simulink model "prelab1"  (R2020a)
settings: Solver=VariableStepAuto  StartTime=0.0  StopTime=10.0  RelTol=1e-3
values from neighbouring files (symbols this model uses):
  backEmfConstant = Kb    (= 0.4173)    [simplified_tf.m]    (also in transferFunctionsDef.m)
  electricalWindingOfMotor = 1/(La*s+Ra)    [simplified_tf.m]    (also in transferFunctionsDef.m)
  mechanicalBlock = 1/(Jeq*s+B)    [simplified_tf.m]    (also in transferFunctionsDef.m)
  motorConstant = Kt    (= 0.72)    [simplified_tf.m]    (also in transferFunctionsDef.m)
  pWMAmplifier = Kvp + Kvi/s    [simplified_tf.m]    (also in transferFunctionsDef.m)
undefined symbols (not defined in the file or in its folder): ElectricalWindingOfMotorDCGain, PWMAmplifierDCgain
libraries: cstblocks x45
settings Model: Creator=brucecui  LastModifiedBy=brucecui

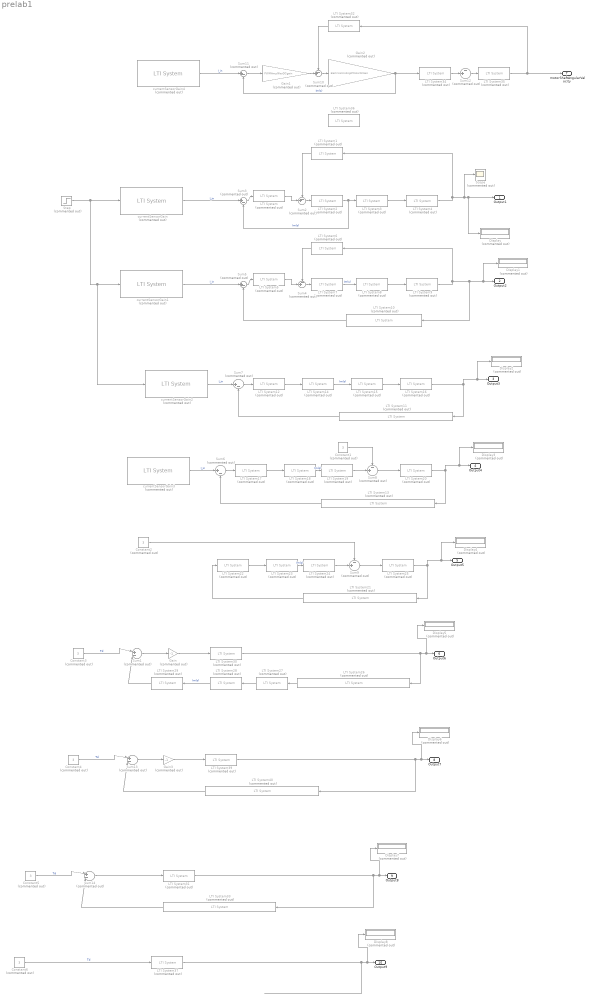
== system prelab1 ==
  Constant{1..6} (6 alike) : Constant  Commented=on  Value=3
  Display{,1..8} (9 alike) : Display  Commented=on
  Gain : Gain  Commented=on  Gain=-1
  Gain1 : Gain  Commented=on  Gain=PWMAmplifierDCgain
  Gain2 : Gain  Commented=on  Gain=ElectricalWindingOfMotorDCGain
  Gain3 : Gain  Commented=on  Gain=-1
  LTI System{,5,12,17} (4 alike) : cstblocks/LTI System  Commented=on  sys=pWMAmplifier  IC=[]
  LTI System{1,6,32,36} (4 alike) : cstblocks/LTI System  Commented=on  sys=backEmfConstant  IC=[]
  LTI System10 : cstblocks/LTI System  Commented=on  sys=1/(motorConstant*mechanicalBlock)  IC=[]
  LTI System{11,13,21,26} (4 alike) : cstblocks/LTI System  Commented=on  sys=1/(motorConstant*mechanicalBlock) + (backEmfConstant/pWMAmplifier)  IC=[]
  LTI System{2,7,14,18,23,28} (6 alike) : cstblocks/LTI System  Commented=on  sys=electricalWindingOfMotor  IC=[]
  LTI System{3,8,15,19,24,29,34} (7 alike) : cstblocks/LTI System  Commented=on  sys=motorConstant  IC=[]
  LTI System{4,9,16,20,25,30,35,39} (8 alike) : cstblocks/LTI System  Commented=on  sys=mechanicalBlock  IC=[]
  LTI System22 : cstblocks/LTI System  Commented=on  sys=-pWMAmplifier  IC=[]
  LTI System27 : cstblocks/LTI System  Commented=on  sys=-pWMAmplifier  IC=[]
  LTI System31 : cstblocks/LTI System  Commented=on  sys=-mechanicalBlock  IC=[]
  LTI System33 : cstblocks/LTI System  Commented=on  sys=(1/(motorConstant*mechanicalBlock) + (backEmfConstant/pWMAmplifier))*motorConstant*electricalWindingOfMotor*(-pWMAmplifier)  IC=[]
  LTI System37 : cstblocks/LTI System  Commented=on  sys=-mechanicalBlock/(1+(-mechanicalBlock)*((1/(motorConstant*mechanicalBlock) + (backEmfConstant/pWMAmplifier))*motorConstant*electricalWindingOfMotor*(-pWMAmplifier)) )  IC=[]
  LTI System40 : cstblocks/LTI System  Commented=on  sys=(1/(motorConstant*mechanicalBlock) + (backEmfConstant/pWMAmplifier))*motorConstant*electricalWindingOfMotor*(-pWMAmplifier)  IC=[]
  Scope : Scope  Commented=on
  Step : Step  Commented=on  Time=0  SampleTime=0
  Sum1 : Sum  Commented=on  Inputs=|+-|
  Sum{2,4,8..10,12} (6 alike) : Sum  Commented=on  Inputs=-+|
  Sum{3,5..7,11} (5 alike) : Sum  Commented=on  Inputs=|+-
  Sum13 : Sum  Commented=on  Inputs=|+-|
  Sum14 : Sum  Commented=on  Inputs=|+-|
  currentSensorGain{,1..4} (5 alike) : cstblocks/LTI System  Commented=on  sys=currentSensorGain  IC=[]
  Output1 : Outport
  Output2 : Outport  Port=2
  Output3 : Outport  Port=3
  Output4 : Outport  Port=4
  Output5 : Outport  Port=5
  Output6 : Outport  Port=6
  motorShaftAngularVelocity : Outport  Port=7
  Output7 : Outport  Port=8
  Output8 : Outport  Port=9
  Output9 : Outport  Port=10
  wires:
  LTI System4/1 -> LTI System1/1, Scope/1, Display/1, Output1/1
  LTI System2/1 -> Sum3/2, LTI System3/1  "Im(s)"
  LTI System/1 -> Sum2/2
  LTI System3/1 -> LTI System4/1
  Sum2/1 -> LTI System2/1
  LTI System1/1 -> Sum2/1
  currentSensorGain/1 -> Sum3/1  "I_in"
  Sum3/1 -> LTI System/1
  currentSensorGain1/1 -> Sum5/1  "I_in"
  LTI System8/1 -> LTI System9/1
  Sum5/1 -> LTI System5/1
  LTI System6/1 -> Sum4/1
  LTI System5/1 -> Sum4/2
  LTI System7/1 -> LTI System8/1  "Im(s)"
  Sum4/1 -> LTI System7/1
  LTI System9/1 -> LTI System6/1, LTI System10/1, Display1/1, Output2/1
  LTI System10/1 -> Sum5/2
  Step/1 -> currentSensorGain2/1, currentSensorGain1/1, currentSensorGain/1
  LTI System11/1 -> Sum7/2
  LTI System14/1 -> LTI System15/1  "Im(s)"
  currentSensorGain2/1 -> Sum7/1  "I_in"
  LTI System15/1 -> LTI System16/1
  Sum7/1 -> LTI System12/1
  LTI System16/1 -> Display2/1, Output3/1, LTI System11/1
  LTI System12/1 -> LTI System14/1
  LTI System20/1 -> Display3/1, Output4/1, LTI System13/1
  LTI System19/1 -> Sum8/2
  LTI System18/1 -> LTI System19/1  "Im(s)"
  LTI System13/1 -> Sum6/2
  currentSensorGain3/1 -> Sum6/1  "I_in"
  Sum6/1 -> LTI System17/1
  LTI System17/1 -> LTI System18/1
  Sum8/1 -> LTI System20/1
  Constant1/1 -> Sum8/1
  LTI System25/1 -> Display4/1, Output5/1, LTI System21/1
  LTI System22/1 -> LTI System23/1
  LTI System21/1 -> LTI System22/1
  LTI System23/1 -> LTI System24/1  "Im(s)"
  Sum9/1 -> LTI System25/1
  LTI System24/1 -> Sum9/2
  Constant2/1 -> Sum9/1
  Constant3/1 -> Sum1/1  "Td"
  LTI System29/1 -> Sum1/2
  LTI System28/1 -> LTI System29/1  "Im(s)"
  Sum1/1 -> Gain/1
  LTI System27/1 -> LTI System28/1
  LTI System26/1 -> LTI System27/1
  LTI System30/1 -> Display5/1, Output6/1, LTI System26/1
  Gain/1 -> LTI System30/1
  currentSensorGain4/1 -> Sum11/1  "I_in"
  Sum10/1 -> Gain2/1
  LTI System35/1 -> LTI System32/1, motorShaftAngularVelocity/1
  Sum11/1 -> Gain1/1
  Gain1/1 -> Sum10/2
  LTI System34/1 -> Sum12/2
  Gain2/1 -> Sum11/2, LTI System34/1  "Im(s)"
  LTI System32/1 -> Sum10/1
  ? -> currentSensorGain4/1  "Voltage Input"
  Sum12/1 -> LTI System35/1
  ? -> Sum12/1  "Td"
  Gain3/1 -> LTI System39/1
  Constant4/1 -> Sum13/1  "Td"
  LTI System39/1 -> LTI System40/1, Display6/1, Output7/1
  Sum13/1 -> Gain3/1
  LTI System40/1 -> Sum13/2
  Constant5/1 -> Sum14/1  "Td"
  LTI System31/1 -> LTI System33/1, Display7/1, Output8/1
  Sum14/1 -> LTI System31/1
  LTI System33/1 -> Sum14/2
  LTI System37/1 -> Display8/1, Output9/1
  Constant6/1 -> LTI System37/1  "Td"
